simulink model "IROS_Stepping_Avoid"  (R2017b)
settings: Solver=ode45  StartTime=0  StopTime=30  FixedStep=0.0005  EnableMultiTasking=on
InitFcn:
  | % Define intial pelvis state
  | pelvisPosition = [0; 0; 1.01];
  | pelvisAngle = [0; 0; 0*pi/2];
  | pelvisVelocity = [0; 0; 0];
  | pelvisRotation = Rotate(pelvisAngle);
  | pelvisAngularVelocity = [0; 0; 0];
  | 
  | % Init Function
  | Initialize_Controller
  | % Define initial motor states
  | figure;
  | motorPositions = testLegIK_Standing;
  | motorVelocities = zeros(10,1);
  | close(gcf);
values from neighbouring files (symbols this model uses):
  N = floor(traj_time/0.1)    [IROS_MPCStep_Walking.m]
undefined symbols (not defined in the file or in its folder): DiagnosticCodes, X, Y, Z
libraries: sm_lib x37, nesl_utility x23, ComponentLibrary x11, CassieLibrary x2
(part 1 of 2)
settings Model: Creator=case  LastModifiedBy=ciscor
settings SolverCC: ZeroCrossControl=DisableAll  InsertRTBMode=Always
settings DataIOCC: SaveOutput=off  SignalLogging=off  DSMLogging=off  SaveTime=off
settings OptimizationCC: DefaultParameterBehavior=Inlined  UseFloatMulNetSlope=on  InlineInvariantSignals=on  EfficientFloat2IntCast=on  LifeSpan=inf  SimCompilerOptimization=on  AccelVerboseBuild=on
settings DebuggingCC: ReadBeforeWriteMsg=DisableAll  WriteAfterWriteMsg=DisableAll  WriteAfterReadMsg=DisableAll  ParameterUnderflowMsg=error  ParameterTunabilityLossMsg=error  UniqueDataStoreMsg=error  AllowSymbolicDim=off  StrictBusMsg=ErrorOnBusTreatedAsVector  SFUnexpectedBacktrackingDiag=warning  SFNoUnconditionalDefaultTransitionDiag=warning  SFExecutionAtInitializationDiag=none
settings HardwareCC: TargetBitPerPointer=64  TargetBitPerSizeT=64  TargetBitPerPtrDiffT=64  TargetLongLongMode=on  TargetIntDivRoundTo=Zero  TargetEndianess=LittleEndian  TargetWordSize=64  TargetHWDeviceType=MATLAB Host  ProdEqTarget=off
settings ModelReferenceCC: EnableParallelModelReferenceBuilds=on  ModelReferenceNumInstancesAllowed=Zero  ModelReferenceMinAlgLoopOccurrences=on  PropagateSignalLabelsOutOfModel=off
settings RTWCC: Description=Generic Real-Time Target  BuildConfiguration=Faster Runs  CheckMdlBeforeBuild=Warning
settings CodeAppCC: GenerateComments=off  SimulinkBlockComments=off
settings GRTTargetCC: MatFileLogging=off  MultiInstanceERTCode=on  CodeInterfacePackaging=Reusable function  SupportNonFinite=off  GenerateAllocFcn=on
settings ConfigComp: CovMetricSettings=dw  CovHtmlReporting=on  CovSaveCumulativeToWorkspaceVar=on  CovSaveSingleToWorkspaceVar=on  CovExternalEMLEnable=off
settings SimscapeCC: SimscapeNormalizeSystem=off
settings DiagnosticsConfigSet: SimMechanicsRigidlyBoundBlock=warning
settings ExplorerConfigSet: InternalSimMechanicsExplorerSettings="<ExplorerConfiguration><canonicalview>default</canonicalview><AnimationSetting><BasePlaybackSpeed>1.0</BasePlaybackSpeed><PlaybackSpeedFactor>1.0</PlaybackSpeedFactor></AnimationSetting><TilePanel><TileInfo><Tiles Columns=\"2\" Count=\"4\" Rows=\"2\"><Column Weight=\"0.4997\"/><Column Weight=\"0.5003\"/><Row Weight=\"0.4994\"/><Row Weight=\"0.5006\"/><Tile Height=\"1\" Width=\"1\" X=\"0\" Y=\"0\"/><Tile Height=\"1\" Width=\"1\" X=\"0\" Y=\"1\"/><Tile Height=\"1\" Width=\"1\" X=\"1\" Y=\"0\"/><Tile Height=\"1\" Width=\"1\" X=\"1\" Y=\"1\"/></Tiles></TileInfo><SceneInfo><SceneViewer><BGColor><R>0.60000002384185791</R><G>0.60000002384185791</G><B>0.60000002384185791</B></BGColor><Camera><DoPerspective>off</DoPerspective><Position><X>0.125259979788625242</X><Y>-35.4589435179607264</Y><Z>0.669495701191679005</Z></Position><Center><X>0.125259979788625242</X><Y>-1.63155540633397322e-07</Y><Z>0.669495701191679005</Z></Center><Up><X>0</X><Y>-0</Y><Z>1</Z></Up><ViewLimDist>1</ViewLimDist><YLim>0.793520828344570717</YLim><XLim>1.30287541410628838</XLim></Camera></SceneViewer><SceneViewer><BGColor><R>0.60000002384185791</R><G>0.60000002384185791</G><B>0.60000002384185791</B></BGColor><Camera><DoPerspective>off</DoPerspective><Position><X>0.335928567731834993</X><Y>-0.127348506171865383</Y><Z>35.6885747346515885</Z></Position><Center><X>0.335928567731834993</X><Y>-0.127348506171865383</Y><Z>0.527048019215854424</Z></Center><Up><X>0</X><Y>1</Y><Z>-0</Z></Up><ViewLimDist>1</ViewLimDist><YLim>1.58989296739346031</YLim><XLim>2.59872639737630617</XLim></Camera></SceneViewer><SceneViewer><BGColor><R>0.60000002384185791</R><G>0.60000002384185791</G><B>0.60000002384185791</B></BGColor><Camera><DoPerspective>off</DoPerspective><Position><X>35.4589435115448453</X><Y>-0.238848601480886658</Y><Z>0.761524082450177775</Z></Position><Center><X>8.0474411845443683e-07</X><Y>-0.238848601480886658</Y><Z>0.761524082450177775</Z></Center><Up><X>-0</X><Y>0</Y><Z>1</Z></Up><ViewLimDist>1</ViewLimDist><YLim>0.773420743950763434</YLim><XLim>1.26987324851375338</XLim></Camera></SceneViewer><SceneViewer><BGColor><R>0.60000002384185791</R><G>0.60000002384185791</G><B>0.60000002384185791</B></BGColor><Camera><DoPerspective>off</DoPerspective><Position><X>21.0273880159162019</X><Y>-19.8053505805593737</Y><Z>20.5055258076376248</Z></Position><Center><X>0.577966597854777331</X><Y>0.644070837502055848</Y><Z>0.0561043895761924039</Z></Center><Up><X>-0.408248290463863073</X><Y>0.408248290463863073</Y><Z>0.816496580927726145</Z></Up><ViewLimDist>1</ViewLimDist><YLim>2.1865649915247185</YLim><XLim>3.57400421260430434</XLim></Camera></SceneViewer></SceneInfo></TilePanel><MechEditorPanel><Cameras><Camera><Id>Camera1</Id><Value><Name>Tracking Camera</Name><NativeCamera><PositionTrackingFeature>Cassie.Cassie_Simulation.World.Tracking_Camera.F</PositionTrackingFeature><CenterTrackingFeature>Cassie.Cassie_Simulation.World.Tracking_Camera_Target.F</CenterTrackingFeature><UpVectorTrackingFeature>Cassie.Cassie_Simulation.World.Tracking_Camera_Target.F</UpVectorTrackingFeature><CenterTrackingOrigin>on</CenterTrackingOrigin><UpVectorTrackingDirection>+Z</UpVectorTrackingDirection></NativeCamera></Value></Camera><Camera><Id>Camera2</Id><Value><Name>Fixed Camera</Name><NativeCamera><PositionTrackingFeature>Cassie.Cassie_Simulation.World.Fixed_Camera.F</PositionTrackingFeature><CenterTrackingFeature>Cassie.Cassie_Simulation.World.Fixed_Camera_Target.F</CenterTrackingFeature><UpVectorTrackingFeature>Cassie.Cassie_Simulation.World.Fixed_Camera_Target.F</UpVectorTrackingFeature><CenterTrackingOrigin>on</CenterTrackingOrigin><UpVectorTrackingDirection>+Z</UpVectorTrackingDirection></NativeCamera></Value></Camera></Cameras><GfxPanelCameraMap/><VideoCreator><PlaybackSpeedRatio>1.0</PlaybackSpeedRatio><FrameRate>60</FrameRate><VideoFormat>MPEG-4</VideoFormat><FrameSize>auto</FrameSize></VideoCreator></MechEditorPanel></ExplorerConfiguration>"

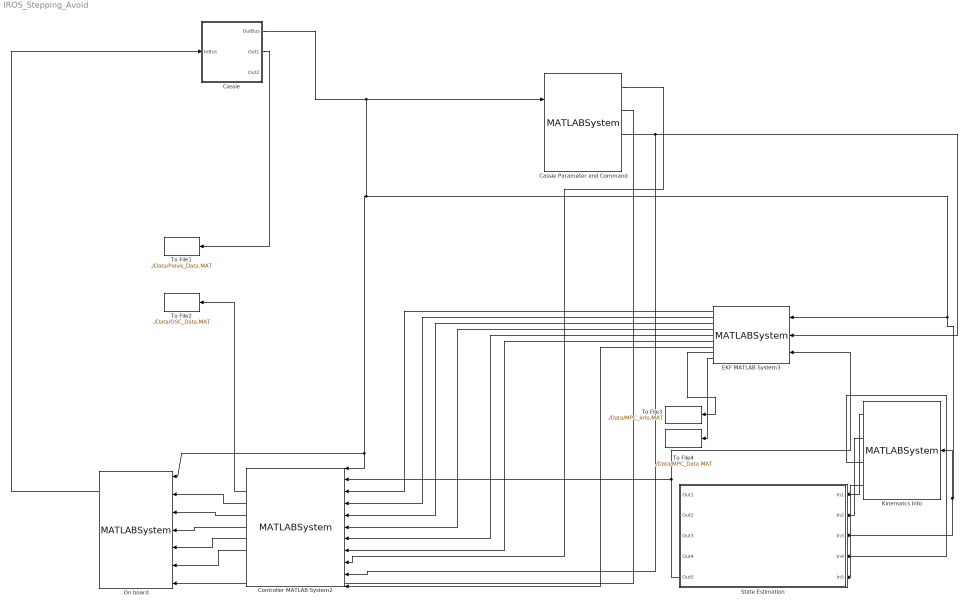
== system IROS_Stepping_Avoid ==
  Cassie : Subsystem  AncestorBlock=CassieLibrary/Simulation/Cassie  InitFcn=|  StartFcn=|  StopFcn=|
      InitFcn=|
      | % Start clock at initialization (used for computing real time performance)
      | initTime = tic;
      | 
      | % Import bus definitions
      | CassieModule.importBuses;
      StartFcn=|
      | % Store build time
      | buildTime = toc(initTime);
      StopFcn=|
      | % Store computation time
      | computationTime = toc(initTime) - buildTime;
      | 
      | % Get simulation time
      | simulationTime = get_param(bdroot, 'SimulationTime');
      | 
      | % Compute real time performance
      | percentRealTime = 100*simulationTime/computationTime;
      | 
      | % Display
      | fprintf('Build time: %0.2f seconds \n', buildTime);
      | fprintf('Simulation time: %0.2f seconds \n', simulationTime);
      | fprintf('Computation time: %0.2f seconds \n', computationTime);
      | fprintf('Performance: %0.2f%% real time \n', percentRealTime);
      mask Display: image('Cassie.png');
  Cassie Parameter and Command : MATLABSystem  System=Cassie_SSDS_Param  is_sim=1  is_IK=0  SimulateUsing=Code generation
      mask Type: Cassie_SSDS_Param
      mask Display:
      | disp('Cassie_SSDS_Param');
      | port_label('output',1,'gain');
      | port_label('output',2,'weight');
      | port_label('output',3,'stepping_command');
      | port_label('output',4,'velocity_command');
  Controller MATLAB System2 : MATLABSystem  System=IROS_MPCStep_Walking  is_sim=1  is_IK=0  SimulateUsing=Code generation
      mask Type: IROS_MPCStep_Walking
      mask Display:
      | disp('IROS_MPCStep_Walking');
      | port_label('input',1,'cassieOutputs');
      | port_label('input',2,'pos_vel_port');
      | port_label('input',3,'pel_pos_traj');
      | port_label('input',4,'pel_vel_traj');
      | port_label('input',5,'pel_acc_traj');
      | port_label('input',6,'contact_traj');
      | port_label('input',7,'contact_switch');
      | port_label('input',8,'traj_time');
      | port_label('input',9,'gains');
      | port_label('input',10,'stepping_command');
      | port_label('input',11,'sec_QP_Data');
      | port_label('output',1,'userInputs');
      | port_label('output',2,'Data');
      | port_label('output',3,'Inertia');
      | port_label('output',4,'Jaco');
      | port_label('output',5,'contact_comd');
      | port_label('output',6,'acc_comd');
      | port_label('output',7,'other_info');
      | port_label('output',8,'states');
      | port_label('output',9,'MPC_Data');
  EKF MATLAB System3 : MATLABSystem  System=IRO_MPCStepAvoid_Traj  is_sim=1  x_obs_int=x_start  SimulateUsing=Code generation
      mask Type: IRO_MPCStepAvoid_Traj
      mask Display:
      | disp('IRO_MPCStepAvoid_Traj');
      | port_label('output',1,'des_pos');
      | port_label('output',2,'des_vel');
      | port_label('output',3,'des_acc');
      | port_label('output',4,'contact');
      | port_label('output',5,'contact_switch');
      | port_label('output',6,'traj_time');
      | port_label('output',7,'sc_Data');
      | port_label('output',8,'MPC_Slack');
      | port_label('output',9,'MPC_Data');
  "Kinematcs Info " : MATLABSystem  System=Kinematics_Info  SimulateUsing=Code generation
      mask Type: Kinematics_Info
      mask Display:
      | disp('Kinematics_Info');
      | port_label('output',1,'lfmp');
      | port_label('output',2,'rfmp');
      | port_label('output',3,'lfmj');
      | port_label('output',4,'rfmj');
  "On board " : MATLABSystem  System=IROS_On_board_QP  is_IK=0  SimulateUsing=Code generation
      mask Type: IROS_On_board_QP
      mask Display: disp('IROS_On_board_QP');
  State Estimation : Subsystem
  To File1 : ToFile  Filename=./Data/Pelvis_Data.MAT  MatrixName=data
  To File2 : ToFile  Filename=./Data/OSC_Data.MAT  MatrixName=data
  To File3 : ToFile  Filename=./Data/MPC_Info.MAT  MatrixName=data
  To File4 : ToFile  Filename=./Data/MPC_Data.MAT  MatrixName=data
  wires:
  Cassie/2(Out1) -> To File1/1
  EKF MATLAB System3/2 -> Controller MATLAB System2/4
  EKF MATLAB System3/3 -> Controller MATLAB System2/5
  EKF MATLAB System3/4 -> Controller MATLAB System2/6
  EKF MATLAB System3/5 -> Controller MATLAB System2/7
  EKF MATLAB System3/1 -> Controller MATLAB System2/3
  Cassie Parameter and Command/3 -> Controller MATLAB System2/10, EKF MATLAB System3/2
  "Kinematcs Info "/1 -> State Estimation/1(In1)
  "Kinematcs Info "/2 -> State Estimation/2(In2)
  "Kinematcs Info "/3 -> State Estimation/4(In4)
  "Kinematcs Info "/4 -> State Estimation/5(In5)
  Cassie Parameter and Command/1 -> Controller MATLAB System2/9
  EKF MATLAB System3/6 -> Controller MATLAB System2/8
  "On board "/1 -> Cassie/1(InBus)
  Cassie Parameter and Command/2 -> "On board "/7
  Cassie/1(OutBus) -> "Kinematcs Info "/1, State Estimation/3(In3), EKF MATLAB System3/1, Controller MATLAB System2/1, "On board "/1, Cassie Parameter and Command/1
  State Estimation/5(Out5) -> EKF MATLAB System3/3, Controller MATLAB System2/2
  Controller MATLAB System2/6 -> "On board "/5
  Controller MATLAB System2/3 -> "On board "/2
  Controller MATLAB System2/4 -> "On board "/3
  Controller MATLAB System2/5 -> "On board "/4
  Controller MATLAB System2/7 -> "On board "/6
  EKF MATLAB System3/7 -> Controller MATLAB System2/11
  EKF MATLAB System3/8 -> To File3/1
  Controller MATLAB System2/2 -> To File2/1
  EKF MATLAB System3/9 -> To File4/1

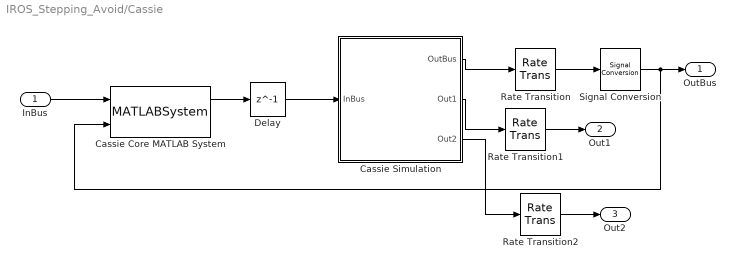
== system IROS_Stepping_Avoid/Cassie ==
  InBus : Inport  OutDataTypeStr=Bus: CassieUserInBus
  Cassie Core MATLAB System : MATLABSystem  System=CassieCoreSim  SimulateUsing=Interpreted execution
      mask Type: CassieCoreSim
      mask Display: disp('CassieCoreSim');
  Cassie Simulation : Subsystem  AncestorBlock=CassieLibrary/Simulation/Cassie Simulation
      mask Display: image('Cassie.png');
  Delay : Delay  DelayLength=1
  Rate Transition : RateTransition  OutPortSampleTime=0.0005
  Rate Transition1 : RateTransition  OutPortSampleTime=0.0005
  Rate Transition2 : RateTransition  OutPortSampleTime=0.0005
  Signal Conversion : SignalConversion  ConversionOutput=Nonvirtual bus  OutDataTypeStr=Bus: CassieOutBus  OverrideOpt=off
  OutBus : Outport  OutDataTypeStr=Bus: CassieOutBus
  Out1 : Outport  Port=2
  Out2 : Outport  Port=3
  wires:
  Signal Conversion/1 -> Cassie Core MATLAB System/2, OutBus/1
  Cassie Simulation/1(OutBus) -> Rate Transition/1
  Rate Transition/1 -> Signal Conversion/1
  Delay/1 -> Cassie Simulation/1(InBus)
  Cassie Core MATLAB System/1 -> Delay/1
  InBus/1 -> Cassie Core MATLAB System/1
  Cassie Simulation/2(Out1) -> Rate Transition1/1
  Rate Transition1/1 -> Out1/1
  Cassie Simulation/3(Out2) -> Rate Transition2/1
  Rate Transition2/1 -> Out2/1

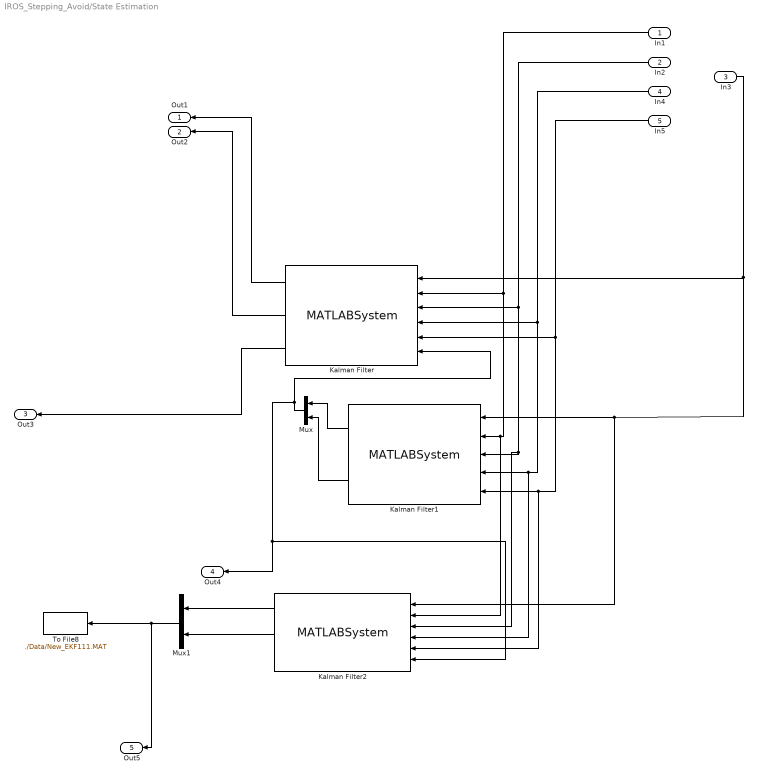
== system IROS_Stepping_Avoid/State Estimation ==
  In1 : Inport
  In2 : Inport  Port=2
  In3 : Inport  Port=3
  In4 : Inport  Port=4
  In5 : Inport  Port=5
  Kalman Filter : MATLABSystem  System=Sim_CassieEKF_Bias  static_bias_initialization=true  ekf_update_enabled=true  enable_kinematic_measurements=true  gyro_bias_init=zeros( 3, 1 )  accel_bias_init=zeros( 3, 1 )  SimulateUsing=Code generation
      mask Type: Sim_CassieEKF_Bias
      mask Display:
      | disp('Sim_CassieEKF_Bias');
      | port_label('input',1,'cassieOutputs');
      | port_label('input',2,'lfm_pos');
      | port_label('input',3,'rfm_pos');
      | port_label('input',4,'lfm_jaco');
      | port_label('input',5,'rfm_jaco');
      | port_label('input',6,'pel_pos_vel');
      | port_label('output',1,'pel_pos_estimation');
      | port_label('output',2,'pel_vel_estimation');
      | port_label('output',3,'other');
  Kalman Filter1 : MATLABSystem  System=Cassie_Kinematic_Es  SimulateUsing=Code generation
      mask Type: Cassie_Kinematic_Es
      mask Display:
      | disp('Cassie_Kinematic_Es');
      | port_label('input',1,'CassieOutput');
      | port_label('input',2,'lfmp');
      | port_label('input',3,'rfmp');
      | port_label('input',4,'lfmj');
      | port_label('input',5,'rfmj');
  Kalman Filter2 : MATLABSystem  System=Sim_CassieEKFDecoupled_BiasV2  static_bias_initialization=true  ekf_update_enabled=true  enable_kinematic_measurements=true  gyro_bias_init=zeros( 3, 1 )  accel_bias_init=zeros( 3, 1 )  SimulateUsing=Code generation
      mask Type: Sim_CassieEKFDecoupled_BiasV2
      mask Display:
      | disp('Sim_CassieEKFDecoupled_BiasV2');
      | port_label('input',1,'cassieOutputs');
      | port_label('input',2,'lfm_pos');
      | port_label('input',3,'rfm_pos');
      | port_label('input',4,'lfm_jaco');
      | port_label('input',5,'rfm_jaco');
      | port_label('input',6,'pel_pos_vel');
      | port_label('output',1,'pel_pos_estimation');
      | port_label('output',2,'pel_vel_estimation');
      | port_label('output',3,'other');
  Mux : Mux  Inputs=2
  Mux1 : Mux  Inputs=2
  To File8 : ToFile  Filename=./Data/New_EKF111.MAT  MatrixName=data
  Out1 : Outport
  Out2 : Outport  Port=2
  Out3 : Outport  Port=3
  Out4 : Outport  Port=4
  Out5 : Outport  Port=5
  wires:
  In1/1 -> Kalman Filter2/2, Kalman Filter1/2, Kalman Filter/2
  Kalman Filter/1 -> Out1/1
  Kalman Filter/2 -> Out2/1
  Kalman Filter1/2 -> Mux/2
  Kalman Filter/3 -> Out3/1
  Mux/1 -> Kalman Filter2/6, Out4/1, Kalman Filter/6
  Kalman Filter1/1 -> Mux/1
  In5/1 -> Kalman Filter/5, Kalman Filter2/5, Kalman Filter1/5
  In2/1 -> Kalman Filter/3, Kalman Filter2/3, Kalman Filter1/3
  In4/1 -> Kalman Filter/4, Kalman Filter2/4, Kalman Filter1/4
  In3/1 -> Kalman Filter2/1, Kalman Filter1/1, Kalman Filter/1
  Kalman Filter2/1 -> Mux1/1
  Kalman Filter2/2 -> Mux1/2
  Mux1/1 -> Out5/1, To File8/1

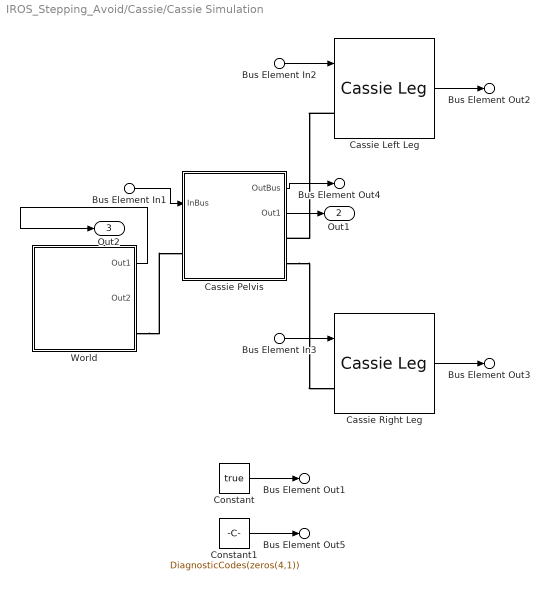
== system IROS_Stepping_Avoid/Cassie/Cassie Simulation ==
  Bus Element In2 : Inport  PortName=InBus  Element=leftLeg
  Bus Element In3 : Inport  PortName=InBus  Element=rightLeg
  Bus Element In1 : Inport  PortName=InBus  Element=pelvis
  Cassie Left Leg : CassieLibrary/Simulation/Cassie Leg  config=Left  motorPositions=motorPositions(1:5)  motorVelocities=motorVelocities(1:5)
      link override Foot Solid: GraphicDiffuseColor=[1.0 1.0 1.0]
      link override Heel Ground Contact: vis_clr="[0.0  1 0.0]"  mu_kinetic=0.7  mu_static=0.9
      link override Heel Ground Contact/Visual PlaBnZ: GraphicDiffuseColor=[1.0 1.0 1.0]  GraphicVisPropType=AdvancedVisualProperties  GraphicAmbientColor=[1.0 1.0 1.0 1.0]
      link override Heel Ground Contact/Visual PlaBpZ: GraphicDiffuseColor=[1.0 1.0 1.0]  GraphicVisPropType=AdvancedVisualProperties  GraphicAmbientColor=[1.0 1.0 1.0 1.0]
      link override Heel Spring Revolute Joint: SpringStiffness=1250
      link override Hip Roll Solid: GraphicDiffuseColor=[1.0 1.0 1.0]
      link override Knee Spring Revolute Joint: SpringStiffness=1500
      link override Shin Solid: GraphicDiffuseColor=[0.8 0.8 0.8]  GraphicOpacity=1
      link override Tarsus Solid: GraphicDiffuseColor=[0.8 0.8 0.8]  GraphicOpacity=1
      link override Toe Ground Contact: vis_clr="[0.0  1 0.0]"  mu_kinetic=0.7  mu_static=0.9
      link override Toe Ground Contact/Visual PlaBnZ: GraphicDiffuseColor=[1.0 1.0 1.0]  GraphicVisPropType=AdvancedVisualProperties  GraphicAmbientColor=[1.0 1.0 1.0 1.0]
      link override Toe Ground Contact/Visual PlaBpZ: GraphicDiffuseColor=[1.0 1.0 1.0]  GraphicVisPropType=AdvancedVisualProperties  GraphicAmbientColor=[1.0 1.0 1.0 1.0]
  Cassie Pelvis : Subsystem  AncestorBlock=CassieLibrary/Simulation/Cassie Pelvis
  Cassie Right Leg : CassieLibrary/Simulation/Cassie Leg  config=Right  motorPositions=motorPositions(6:10)  motorVelocities=motorVelocities(6:10)
      link override Foot Solid: GraphicDiffuseColor=[1.0 1.0 1.0]
      link override Heel Ground Contact: vis_clr=[0 1 0]  mu_kinetic=0.7  mu_static=0.9
      link override Heel Ground Contact/Visual PlaBnZ: GraphicDiffuseColor=vis_clr
      link override Heel Ground Contact/Visual PlaBpZ: GraphicDiffuseColor=vis_clr
      link override Heel Spring Revolute Joint: SpringStiffness=1250
      link override Hip Roll Solid: GraphicDiffuseColor=[1.0 1.0 1.0]
      link override Knee Spring Revolute Joint: SpringStiffness=1500
      link override Shin Solid: GraphicDiffuseColor=[0.7529412 0.7529412 0.7529412]
      link override Tarsus Solid: GraphicDiffuseColor=[0.7529412 0.7529412 0.7529412]
      link override Toe Ground Contact: vis_clr=[0 1 0]  mu_kinetic=0.7  mu_static=0.9
      link override Toe Ground Contact/Visual PlaBnZ: GraphicDiffuseColor=vis_clr
      link override Toe Ground Contact/Visual PlaBpZ: GraphicDiffuseColor=vis_clr
  Constant : Constant  Value=true
  Constant1 : Constant  Value=DiagnosticCodes(zeros(4,1))
  World : Subsystem  AncestorBlock=ComponentLibrary/Simulation/World
  Bus Element Out4 : Outport  PortName=OutBus  Element=pelvis
  Bus Element Out2 : Outport  PortName=OutBus  Element=leftLeg
  Bus Element Out3 : Outport  PortName=OutBus  Element=rightLeg
  Bus Element Out1 : Outport  PortName=OutBus  Element=isCalibrated
  Bus Element Out5 : Outport  PortName=OutBus  Element=messages
  Out1 : Outport  Port=2
  Out2 : Outport  Port=3
  wires:
  Constant1/1 -> Bus Element Out5/1
  Constant/1 -> Bus Element Out1/1
  Bus Element In1/1 -> Cassie Pelvis/1(InBus)
  Cassie Right Leg/1 -> Bus Element Out3/1
  Bus Element In2/1 -> Cassie Left Leg/1
  Cassie Left Leg/1 -> Bus Element Out2/1
  Bus Element In3/1 -> Cassie Right Leg/1
  Cassie Pelvis/1(OutBus) -> Bus Element Out4/1
  Cassie Pelvis/2(Out1) -> Out1/1
  World/1(Out1) -> Out2/1
  connections:
  World/RConn1 -- Cassie Pelvis/LConn1
  Cassie Left Leg/LConn1 -- Cassie Pelvis/RConn1
  Cassie Pelvis/RConn2 -- Cassie Right Leg/LConn1

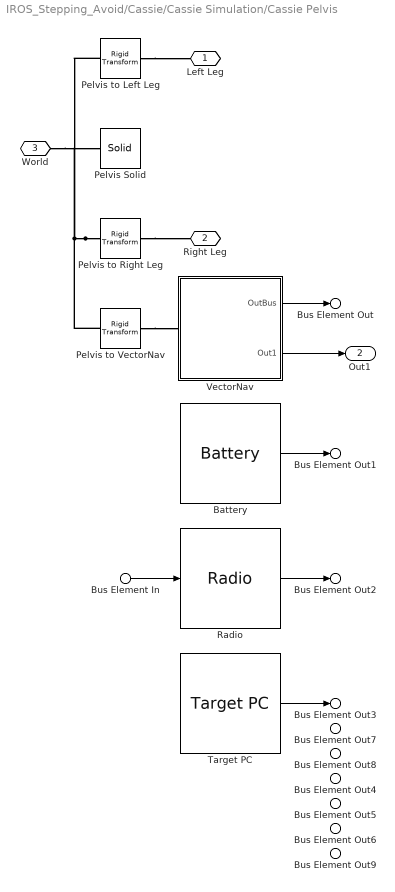
== system IROS_Stepping_Avoid/Cassie/Cassie Simulation/Cassie Pelvis ==
  Bus Element In : Inport  PortName=InBus  Element=radio
  Battery : ComponentLibrary/Simulation/Battery  SystemSampleTime=-1
  Pelvis Solid : sm_lib/Body Elements/Solid  InertiaType=Custom  Mass=10.33  MassUnits=kg  CenterOfMass=[0.05066 0.000346 0.02841]  CenterOfMassUnits=m  MomentsOfInertia=[0.085821 0.049222 0.08626]  MomentsOfInertiaUnits=kg*m^2  ProductsOfInertia=[1.276e-05 -0.00016022 -0.000414]  ProductsOfInertiaUnits=kg*m^2  DensityBased=on  Density=1000  DensityUnits=kg/(m^3)  DoExposeReferenceFrame=on  SerializedFrames=<Frames/>  GraphicType=FromGeometry  MarkerShape=Sphere  MarkerSize=10  GraphicVisPropType=SimpleVisualProperties  GraphicDiffuseColor=[0.6 0.6 0.6]  GraphicSpecularColor=[0.5 0.5 0.5 1.0]  GraphicAmbientColor=[0.5 0.5 0.5 1.0]  GraphicEmissiveColor=[0.5 0.5 0.5 1.0]  GraphicShininess=75  GraphicOpacity=1.0  GeometryShape=FromFile  RectangleSize=[1 1]  RectangleSizeUnits=m  BrickDimensions=[1 1 1]  BrickDimensionUnits=m  CylinderRadius=1  CylinderRadiusUnits=m  CylinderLength=1  CylinderLengthUnits=m  SphereRadius=1  SphereRadiusUnits=m  EllipsoidRadii=[1 1 1]  EllipsoidRadiiUnits=m  ExtrusionCrossSection=[1 1; -1 1; -1 -1; 1 -1]  ExtrusionCrossSectionUnits=m  ExtrusionLength=1  ExtrusionLengthUnits=m  PolygonNumSides=3  PolygonOuterRadius=1  PolygonOuterRadiusUnits=m  ExtGeomFileType=STL  ExtGeomFileName=cassie-pelvis.stl  ExtGeomFileUnits=m  RevolutionCrossSection=[1 1; 1 -1; 2 -1; 2 1]  RevolutionCrossSectionUnits=m  RevolutionExtent=Full  RevolutionAngle=180  RevolutionAngleUnits=deg
  Pelvis to Left Leg : sm_lib/Frames and Transforms/Rigid Transform  TranslationMethod=Cartesian  TranslationStandardOffset=0  TranslationLengthUnit=m  TranslationStandardAxis=+Z  TranslationCartesianOffset=[0.021, 0.135, 0]  TranslationROffset=0  TranslationROffsetUnits=m  TranslationZOffset=0  TranslationZOffsetUnits=m  TranslationThetaOffset=0  TranslationThetaOffsetUnits=deg  RotationMethod=RotationMatrix  RotationAngleUnits=deg  RotationStandardAxis=+Z  RotationAngle=0.0  RotationArbitraryAxis=[0 0 1]  FollAlignAxisA=+X  BaseAlignAxisA=+Y  FollAlignAxisB=+Y  BaseAlignAxisB=+Z  RotationSequenceAxes=FollowerAxes  RotationSequence=XYX  RotationSequenceAngles=[0 0 0]  RotationSequenceAnglesUnits=deg  RotationMatrix=[0, 0, 1; 0, 1, 0; -1, 0, 0]
  Pelvis to Right Leg : sm_lib/Frames and Transforms/Rigid Transform  TranslationMethod=Cartesian  TranslationStandardOffset=0  TranslationLengthUnit=m  TranslationStandardAxis=+Z  TranslationCartesianOffset=[0.021, -0.135, 0]  TranslationROffset=0  TranslationROffsetUnits=m  TranslationZOffset=0  TranslationZOffsetUnits=m  TranslationThetaOffset=0  TranslationThetaOffsetUnits=deg  RotationMethod=RotationMatrix  RotationAngleUnits=deg  RotationStandardAxis=+Z  RotationAngle=0.0  RotationArbitraryAxis=[0 0 1]  FollAlignAxisA=+X  BaseAlignAxisA=+Y  FollAlignAxisB=+Y  BaseAlignAxisB=+Z  RotationSequenceAxes=FollowerAxes  RotationSequence=XYX  RotationSequenceAngles=[0 0 0]  RotationSequenceAnglesUnits=deg  RotationMatrix=[0, 0, 1; 0, 1, 0; -1, 0, 0]
  Pelvis to VectorNav : sm_lib/Frames and Transforms/Rigid Transform  TranslationMethod=Cartesian  TranslationStandardOffset=0  TranslationLengthUnit=cm  TranslationStandardAxis=+Z  TranslationCartesianOffset=[3.155 0 -7.996]  TranslationROffset=0  TranslationROffsetUnits=m  TranslationZOffset=0  TranslationZOffsetUnits=m  TranslationThetaOffset=0  TranslationThetaOffsetUnits=deg  RotationMethod=RotationSequence  RotationAngleUnits=deg  RotationStandardAxis=+Z  RotationAngle=0.0  RotationArbitraryAxis=[0 0 1]  FollAlignAxisA=+X  BaseAlignAxisA=+Y  FollAlignAxisB=+Y  BaseAlignAxisB=+Z  RotationSequenceAxes=FollowerAxes  RotationSequence=ZYX  RotationSequenceAngles=[0 0 180]  RotationSequenceAnglesUnits=deg  RotationMatrix=[1 0 0; 0 1 0; 0 0 1]
  Radio : ComponentLibrary/Simulation/Radio  SystemSampleTime=-1
  Target PC : ComponentLibrary/Simulation/Target PC  SystemSampleTime=-1
  VectorNav : Subsystem  AncestorBlock=ComponentLibrary/Simulation/VectorNav  mask{preRotationMatrix=[1, 0, 0; 0, -1, 0; 0, 0, -1], postRotationMatrix=[1, 0, 0; 0, -1, 0; 0, 0, -1]}
      mask prompts: preRotationMatrix "Pre Rotation Matrix:"; postRotationMatrix "Post Rotation Matrix"
      mask Display: image('VectorNav.png');
  Left Leg : PMIOPort  Port=1  Side=Right
  Right Leg : PMIOPort  Port=2  Side=Right
  World : PMIOPort  Port=3  Side=Left
  Bus Element Out3 : Outport  PortName=OutBus  Element=targetPc
  Bus Element Out1 : Outport  PortName=OutBus  Element=battery
  Bus Element Out2 : Outport  PortName=OutBus  Element=radio
  Bus Element Out : Outport  PortName=OutBus  Element=vectorNav
  Bus Element Out7 : Outport  PortName=OutBus  Element=medullaCounter
  Bus Element Out8 : Outport  PortName=OutBus  Element=medullaCpuLoad
  Bus Element Out4 : Outport  PortName=OutBus  Element=bleederState
  Bus Element Out5 : Outport  PortName=OutBus  Element=leftReedSwitchState
  Bus Element Out6 : Outport  PortName=OutBus  Element=rightReedSwitchState
  Bus Element Out9 : Outport  PortName=OutBus  Element=vtmTemperature
  Out1 : Outport  Port=2
  wires:
  Target PC/1 -> Bus Element Out3/1
  Bus Element In/1 -> Radio/1
  Radio/1 -> Bus Element Out2/1
  Battery/1 -> Bus Element Out1/1
  VectorNav/1(OutBus) -> Bus Element Out/1
  VectorNav/2(Out1) -> Out1/1
  connections:
  Pelvis to VectorNav/RConn1 -- VectorNav/LConn1
  Pelvis to Right Leg/LConn1 -- Pelvis to VectorNav/LConn1 -- World/RConn1 -- Pelvis to Left Leg/LConn1 -- Pelvis Solid/RConn1
  Pelvis to Left Leg/RConn1 -- Left Leg/RConn1
  Pelvis to Right Leg/RConn1 -- Right Leg/RConn1
